simulink model "engineModelF16"  (R2024a)
settings: configuration reference "standardSILConfiguraitonParams" (kept outside this file)
undefined symbols (not defined in the file): engineDataF16, lbf2N, m2ft, parameters, stepSize_s
libraries: simulink x10
settings Model: Creator=jerem  LastModifiedBy=jerem
settings ConfigSetRef: SourceName=standardSILConfiguraitonParams  SourceLocation=Base Workspace

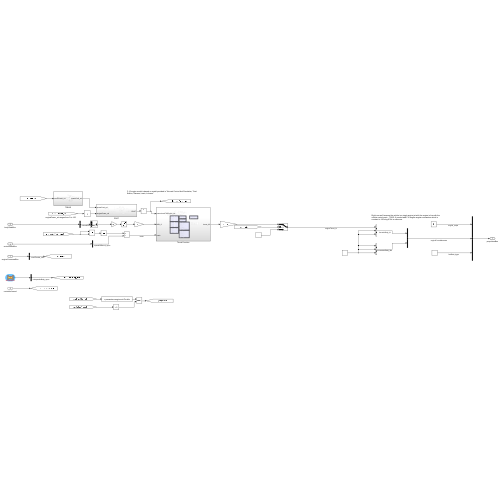
[thumbnail: Simulink's stored preview of the top-level diagram]
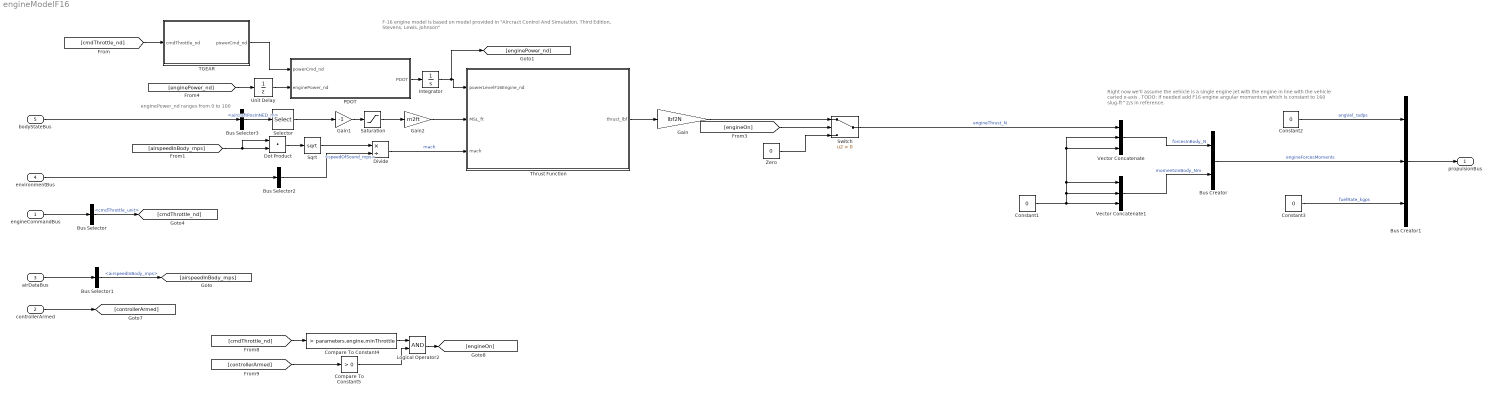
== system engineModelF16 ==
  note: enginePower_nd ranges from 0 to 100
  note: F-16 engine model is based on model provided in "Aircract Control And Simulation, Third Edition, Stevens, Lewis, Johnson"
  note: Right now we'll assume the vehicle is a single engine jet with the engine in line with the vehicle caried x-axis . TODO: If needed add F16 engine angular momentum which is constant to 160 slug-ft^2/s in reference.
  engineCommandBus : Inport  OutDataTypeStr=Bus: EngineCommandBus
  controllerArmed : Inport  Port=2
  airDataBus : Inport  Port=3  OutDataTypeStr=Bus: AirDataBus
  environmentBus : Inport  Port=4  OutDataTypeStr=Bus: EnvironmentBus
  bodyStateBus : Inport  Port=5  OutDataTypeStr=Bus: BodyStateBus
  Bus Creator : BusCreator  Inputs=2
  Bus Creator1 : BusCreator  Inputs=3  OutDataTypeStr=Bus: PropulsionBus
  Bus Selector : BusSelector  OutputSignals=cmdThrottle_unit
  Bus Selector1 : BusSelector  OutputSignals=airspeedInBody_mps
  Bus Selector2 : BusSelector  OutputSignals=AirEnvironment.speedOfSound_mps
  Bus Selector3 : BusSelector  OutputSignals=aircraftPosInNED_m
  Compare To Constant4 : simulink/Logic and Bit Operations/Compare To Constant  relop=>  const=parameters.engine.minThrottle  OutDataTypeStr=boolean
  Compare To Constant5 : simulink/Logic and Bit Operations/Compare To Constant  relop=>  const=0  OutDataTypeStr=boolean
  Constant1 : Constant  Value=0  SampleTime=stepSize_s
  Constant2 : Constant  Value=0  SampleTime=stepSize_s
  Constant3 : Constant  Value=0  SampleTime=stepSize_s
  Divide : Product  Inputs=*/
  Dot Product : DotProduct  OutDataTypeStr=Inherit: Inherit via internal rule
  Gain : Gain  Gain=lbf2N
  Gain1 : Gain  Gain=-1
  Gain2 : Gain  Gain=m2ft
  Integrator : Integrator
  Logical Operator2 : Logic  AllPortsSameDT=off  OutDataTypeStr=boolean
  PDOT : Subsystem
  Saturation : Saturate  UpperLimit=850000  LowerLimit=-1000
  Selector : Selector  InputPortWidth=3  IndexOptions=Index vector (dialog)  Indices=3  OutputSizes=1
  Sqrt : Sqrt
  Switch : Switch  Criteria=u2 > Threshold  SaturateOnIntegerOverflow=off  InputSameDT=off
  TGEAR : Subsystem
  Thrust Function : Subsystem
  Unit Delay : UnitDelay  SampleTime=-1  HasFrameUpgradeWarning=on
  Vector Concatenate : Concatenate  NumInputs=3
  Vector Concatenate1 : Concatenate  NumInputs=3
  Zero : Constant  Value=0  OutDataTypeStr=Inherit: Inherit via back propagation  SampleTime=stepSize_s
  propulsionBus : Outport  OutDataTypeStr=Bus: PropulsionBus
  wires:
  Thrust Function/1(thrust_lbf) -> Gain/1
  Constant1/1 -> Vector Concatenate1/3, Vector Concatenate1/2, Vector Concatenate1/1, Vector Concatenate/3, Vector Concatenate/2
  Vector Concatenate/1 -> Bus Creator/1  "forcesInBody_N"
  Vector Concatenate1/1 -> Bus Creator/2  "momentsInBody_Nm"
  Bus Creator/1 -> Bus Creator1/2  "engineForcesMoments"
  Bus Creator1/1 -> propulsionBus/1
  Constant2/1 -> Bus Creator1/1  "angVel_radps"
  Constant3/1 -> Bus Creator1/3  "fuelRate_kgps"
  Bus Selector/1 -> [cmdThrottle_nd]  "<cmdThrottle_unit>"
  [cmdThrottle_nd] -> Compare To Constant4/1
  engineCommandBus/1 -> Bus Selector/1
  Logical Operator2/1 -> [engineOn]
  controllerArmed/1 -> [controllerArmed]
  airDataBus/1 -> Bus Selector1/1
  Compare To Constant4/1 -> Logical Operator2/1
  Compare To Constant5/1 -> Logical Operator2/2
  [controllerArmed] -> Compare To Constant5/1
  Bus Selector1/1 -> [airspeedInBody_mps]  "<airspeedInBody_mps>"
  Divide/1 -> Thrust Function/3(mach)  "mach"
  environmentBus/1 -> Bus Selector2/1
  Bus Selector2/1 -> Divide/2  "<speedOfSound_mps>"
  bodyStateBus/1 -> Bus Selector3/1
  Bus Selector3/1 -> Selector/1  "<aircraftPosInNED_m>"
  Gain1/1 -> Saturation/1
  Gain2/1 -> Thrust Function/2(MSL_ft)
  Saturation/1 -> Gain2/1
  Selector/1 -> Gain1/1
  [airspeedInBody_mps] -> Dot Product/1, Dot Product/2
  Dot Product/1 -> Sqrt/1
  Sqrt/1 -> Divide/1
  [enginePower_nd] -> Unit Delay/1
  Gain/1 -> Switch/1
  Zero/1 -> Switch/3
  Switch/1 -> Vector Concatenate/1  "engineThrust_N"
  [engineOn] -> Switch/2
  PDOT/1(PDOT) -> Integrator/1
  Integrator/1 -> [enginePower_nd], Thrust Function/1(powerLevelF16Engine_nd)
  Unit Delay/1 -> PDOT/2(enginePower_nd)
  [cmdThrottle_nd] -> TGEAR/1(cmdThrottle_nd)
  TGEAR/1(powerCmd_nd) -> PDOT/1(powerCmd_nd)

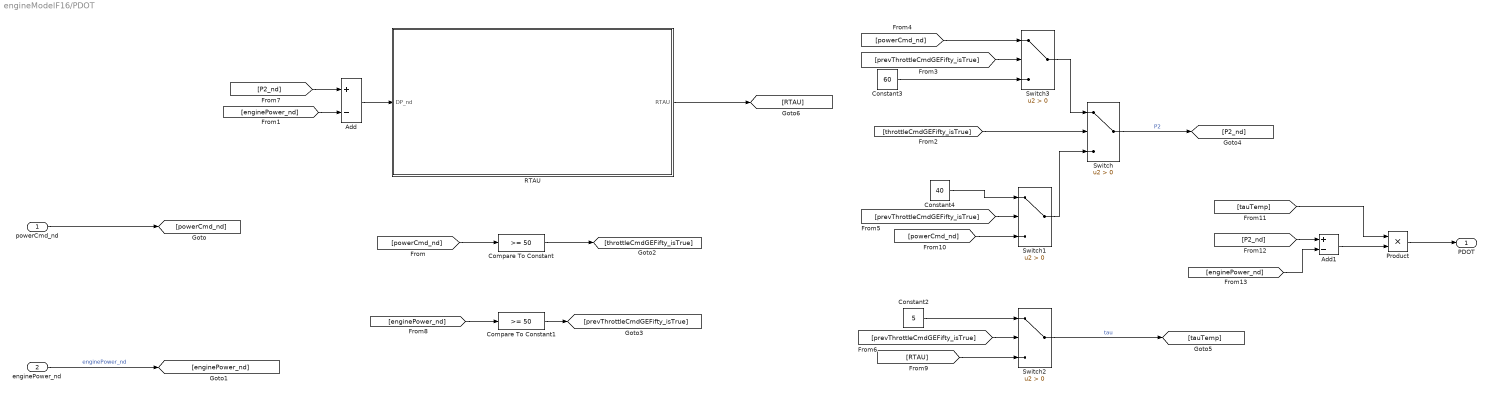
== system engineModelF16/PDOT ==
  powerCmd_nd : Inport
  enginePower_nd : Inport  Port=2
  Add : Sum  Inputs=+-
  Add1 : Sum  Inputs=+-
  Compare To Constant : simulink/Logic and Bit Operations/Compare To Constant  relop=>=  const=50  OutDataTypeStr=boolean
  Compare To Constant1 : simulink/Logic and Bit Operations/Compare To Constant  relop=>=  const=50  OutDataTypeStr=boolean
  Constant2 : Constant  Value=5
  Constant3 : Constant  Value=60
  Constant4 : Constant  Value=40
  Product : Product
  RTAU : Subsystem
  Switch{,1..3} (4 alike) : Switch  Criteria=u2 > Threshold  SaturateOnIntegerOverflow=off  InputSameDT=off
  PDOT : Outport
  wires:
  powerCmd_nd/1 -> [powerCmd_nd]
  enginePower_nd/1 -> [enginePower_nd]  "enginePower_nd"
  [powerCmd_nd] -> Compare To Constant/1
  Compare To Constant/1 -> [throttleCmdGEFifty_isTrue]
  [enginePower_nd] -> Compare To Constant1/1
  Compare To Constant1/1 -> [prevThrottleCmdGEFifty_isTrue]
  [prevThrottleCmdGEFifty_isTrue] -> Switch3/2
  [throttleCmdGEFifty_isTrue] -> Switch/2
  Switch/1 -> [P2_nd]  "P2"
  [prevThrottleCmdGEFifty_isTrue] -> Switch2/2
  Switch2/1 -> [tauTemp]  "tau"
  [P2_nd] -> Add/1
  [enginePower_nd] -> Add/2
  Add/1 -> RTAU/1(DP_nd)
  RTAU/1(RTAU) -> [RTAU]
  Constant2/1 -> Switch2/1
  [RTAU] -> Switch2/3
  [powerCmd_nd] -> Switch3/1
  Switch3/1 -> Switch/1
  Constant3/1 -> Switch3/3
  Switch1/1 -> Switch/3
  [prevThrottleCmdGEFifty_isTrue] -> Switch1/2
  Constant4/1 -> Switch1/1
  [powerCmd_nd] -> Switch1/3
  [P2_nd] -> Add1/1
  [enginePower_nd] -> Add1/2
  Add1/1 -> Product/2
  [tauTemp] -> Product/1
  Product/1 -> PDOT/1

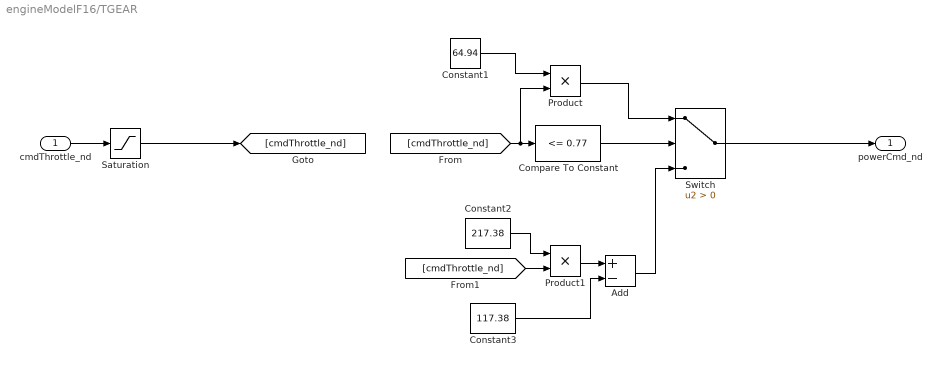
== system engineModelF16/TGEAR ==
  cmdThrottle_nd : Inport
  Add : Sum  Inputs=+-
  Compare To Constant : simulink/Logic and Bit Operations/Compare To Constant  relop=<=  const=0.77  OutDataTypeStr=boolean
  Constant1 : Constant  Value=64.94
  Constant2 : Constant  Value=217.38
  Constant3 : Constant  Value=117.38
  Product : Product
  Product1 : Product
  Saturation : Saturate  UpperLimit=1  LowerLimit=0
  Switch : Switch  Criteria=u2 > Threshold  SaturateOnIntegerOverflow=off  InputSameDT=off
  powerCmd_nd : Outport
  wires:
  cmdThrottle_nd/1 -> Saturation/1
  [cmdThrottle_nd] -> Compare To Constant/1, Product/2
  Compare To Constant/1 -> Switch/2
  Product/1 -> Switch/1
  Constant1/1 -> Product/1
  [cmdThrottle_nd] -> Product1/2
  Constant2/1 -> Product1/1
  Product1/1 -> Add/1
  Constant3/1 -> Add/2
  Add/1 -> Switch/3
  Switch/1 -> powerCmd_nd/1
  Saturation/1 -> [cmdThrottle_nd]

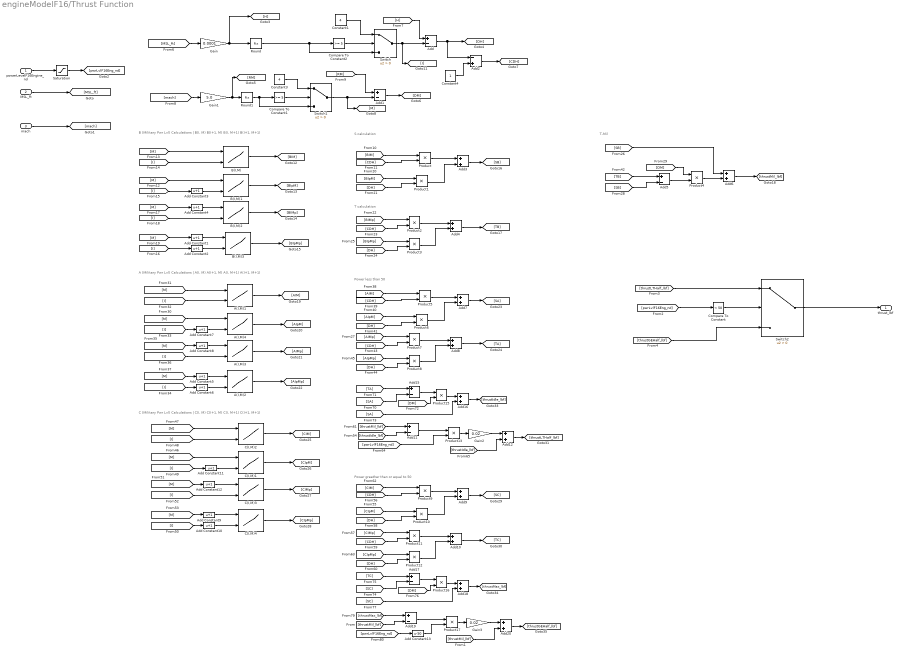
== system engineModelF16/Thrust Function ==
  note: S calculation
  note: B (Military Pwr Lvl) Calculations | B(I, M) B(I+1, M) B(I, M+1) B(I+1, M+1)
  note: T calculation
  note: T-Mil
  note: Power less than 50
  note: A (Military Pwr Lvl) Calculations | A(I, M) A(I+1, M) A(I, M+1) A(I+1, M+1)
  note: C (Military Pwr Lvl) Calculations | C(I, M) C(I+1, M) C(I, M+1) C(I+1, M+1)
  note: Power greather than or equal to 50
  powerLevelF16Engine_nd : Inport  OutDataTypeStr=double
  MSL_ft : Inport  Port=2
  mach : Inport  Port=3
  A(I,M){1..4} (4 alike) : Lookup_n-D  BreakpointsForDimension1=engineDataF16.machBkpts  BreakpointsForDimension2=engineDataF16.altitudeBkpts_ft  Table=engineDataF16.thrustIdle_lbf  ExtrapMethod=Clip  DiagnosticForOutOfRangeInput=Warning  InternalRulePriority=Speed  RndMeth=Simplest
      settings: InputPortMap=u0,u1
  Add{,1,5,11,15,17,19} (7 alike) : Sum  Inputs=+-
  Add Constant{1..12} (12 alike) : Bias  Bias=1  SaturateOnIntegerOverflow=off
  Add Constant13 : Bias  Bias=-50  SaturateOnIntegerOverflow=off
  Add{3..4,6..10,12,16,18,20} (11 alike) : Sum
  Add2 : Sum  Inputs=-+
  B(I,M){,1..3} (4 alike) : Lookup_n-D  BreakpointsForDimension1=engineDataF16.machBkpts  BreakpointsForDimension2=engineDataF16.altitudeBkpts_ft  Table=engineDataF16.thrustMilitary_lbf  ExtrapMethod=Clip  DiagnosticForOutOfRangeInput=Warning  InternalRulePriority=Speed  RndMeth=Simplest
      settings: InputPortMap=u0,u1
  C(I,M){1..4} (4 alike) : Lookup_n-D  BreakpointsForDimension1=engineDataF16.machBkpts  BreakpointsForDimension2=engineDataF16.altitudeBkpts_ft  Table=engineDataF16.thrustMax_lbf  ExtrapMethod=Clip  DiagnosticForOutOfRangeInput=Warning  InternalRulePriority=Speed  RndMeth=Simplest
      settings: InputPortMap=u0,u1
  Compare To Constant : simulink/Logic and Bit Operations/Compare To Constant  relop=<  const=50  OutDataTypeStr=boolean
  Compare To Constant1 : simulink/Logic and Bit Operations/Compare To Constant  relop=>=  const=5  OutDataTypeStr=boolean
  Compare To Constant2 : simulink/Logic and Bit Operations/Compare To Constant  relop=>=  const=5  OutDataTypeStr=boolean
  Constant1 : Constant  Value=4
  Constant3 : Constant  Value=4
  Constant4 : Constant
  Gain : Gain  Gain=0.0001
  Gain1 : Gain  Gain=5.0
  Gain2 : Gain  Gain=0.02
  Gain3 : Gain  Gain=0.02
  Product{,1..13,15..17} (17 alike) : Product
  Round : Rounding  Operator=fix
  Round1 : Rounding  Operator=fix
  Saturation : Saturate  UpperLimit=100  LowerLimit=0
  Switch : Switch  Criteria=u2 > Threshold  SaturateOnIntegerOverflow=off  InputSameDT=off
  Switch1 : Switch  Criteria=u2 > Threshold  SaturateOnIntegerOverflow=off  InputSameDT=off
  Switch2 : Switch  Criteria=u2 > Threshold  SaturateOnIntegerOverflow=off  InputSameDT=off
  thrust_lbf : Outport
  wires:
  powerLevelF16Engine_nd/1 -> Saturation/1
  MSL_ft/1 -> [MSL_ft]
  mach/1 -> [mach]
  [MSL_ft] -> Gain/1
  Gain/1 -> [H], Round/1
  Round/1 -> Compare To Constant2/1, Switch/3
  Compare To Constant2/1 -> Switch/2
  Constant1/1 -> Switch/1
  [H] -> Add/1
  Switch/1 -> [I], Add/2
  Add/1 -> Add2/1, [DH]
  [mach] -> Gain1/1
  Round1/1 -> Compare To Constant1/1, Switch1/3
  Compare To Constant1/1 -> Switch1/2
  Constant3/1 -> Switch1/1
  Gain1/1 -> [RM], Round1/1
  Switch1/1 -> [M], Add1/2
  [RM] -> Add1/1
  Add1/1 -> [DM]
  Constant4/1 -> Add2/2
  Add2/1 -> [CDH]
  [BIM] -> Product/1
  [CDH] -> Product/2
  Product/1 -> Add3/1
  [I] -> Add Constant3/1
  [M] -> Add Constant4/1
  [I] -> Add Constant2/1
  [M] -> Add Constant1/1
  B(I,M)/1 -> [BIM]
  B(I,M)1/1 -> [BIpM]
  B(I,M)2/1 -> [BIMp]
  B(I,M)3/1 -> [BIpMp]
  [BIpM] -> Product1/1
  [DH] -> Product1/2
  Product1/1 -> Add3/2
  Add3/1 -> [SB]
  [BIMp] -> Product2/1
  [CDH] -> Product2/2
  Product2/1 -> Add4/1
  [DH] -> Product3/2
  [BIpMp] -> Product3/1
  Product3/1 -> Add4/2
  Add4/1 -> [TB]
  [TB] -> Add5/1
  [SB] -> Add5/2
  Add5/1 -> Product4/2
  [DM] -> Product4/1
  Product4/1 -> Add6/2
  [SB] -> Add6/1
  Add6/1 -> [thrustMil_lbf]
  [M] -> Add Constant8/1
  [I] -> Add Constant6/1
  A(I,M)3/1 -> [AIMp]
  [I] -> Add Constant7/1
  A(I,M)2/1 -> [AIpMp]
  [M] -> Add Constant5/1
  A(I,M)1/1 -> [AIM]
  A(I,M)4/1 -> [AIpM]
  [CDH] -> Product5/2
  Product5/1 -> Add7/1
  [AIM] -> Product5/1
  [DH] -> Product6/2
  Product6/1 -> Add7/2
  [AIpM] -> Product6/1
  Add7/1 -> [SA]
  [DH] -> Product8/2
  [AIpMp] -> Product8/1
  Product7/1 -> Add8/1
  [AIMp] -> Product7/1
  Product8/1 -> Add8/2
  [CDH] -> Product7/2
  Add8/1 -> [TA]
  C(I,M)4/1 -> [CIpMp]
  C(I,M)1/1 -> [CIpM]
  [M] -> Add Constant9/1
  C(I,M)2/1 -> [CIM]
  C(I,M)3/1 -> [CIMp]
  [M] -> Add Constant12/1
  [I] -> Add Constant11/1
  [I] -> Add Constant10/1
  Product10/1 -> Add9/2
  Add9/1 -> [SC]
  [CIpM] -> Product10/1
  Product11/1 -> Add10/1
  Add10/1 -> [TC]
  Product12/1 -> Add10/2
  [DH] -> Product12/2
  [DH] -> Product10/2
  [CIM] -> Product9/1
  [CIMp] -> Product11/1
  Product9/1 -> Add9/1
  [CIpMp] -> Product12/1
  [CDH] -> Product9/2
  [CDH] -> Product11/2
  [TA] -> Add15/1
  [SA] -> Add15/2
  Add15/1 -> Product15/1
  [DM] -> Product15/2
  Product15/1 -> Add16/1
  [SA] -> Add16/2
  Add16/1 -> [thrustIdle_lbf]
  [thrustMil_lbf] -> Add11/1
  [thrustIdle_lbf] -> Add11/2
  Add11/1 -> Product13/1
  [pwrLvlF16Eng_nd] -> Product13/2
  Product13/1 -> Gain2/1
  Gain2/1 -> Add12/1
  [thrustIdle_lbf] -> Add12/2
  Add12/1 -> [thrustLTHalf_lbf]
  Add17/1 -> Product16/1
  [DM] -> Product16/2
  Add18/1 -> [thrustMax_lbf]
  [TC] -> Add17/1
  [SC] -> Add18/2
  [SC] -> Add17/2
  Product16/1 -> Add18/1
  [thrustMil_lbf] -> Add19/2
  Add20/1 -> [thrustGEHalf_lbf]
  [thrustMil_lbf] -> Add20/2
  Gain3/1 -> Add20/1
  [pwrLvlF16Eng_nd] -> Add Constant13/1
  Add19/1 -> Product17/1
  Product17/1 -> Gain3/1
  [thrustMax_lbf] -> Add19/1
  Add Constant13/1 -> Product17/2
  [pwrLvlF16Eng_nd] -> Compare To Constant/1
  Saturation/1 -> [pwrLvlF16Eng_nd]
  Compare To Constant/1 -> Switch2/2
  [thrustGEHalf_lbf] -> Switch2/3
  [thrustLTHalf_lbf] -> Switch2/1
  Switch2/1 -> thrust_lbf/1
  [M] -> B(I,M)/1
  [I] -> B(I,M)/2
  Add Constant3/1 -> B(I,M)1/2
  [M] -> B(I,M)1/1
  Add Constant4/1 -> B(I,M)2/1
  [I] -> B(I,M)2/2
  Add Constant2/1 -> B(I,M)3/2
  Add Constant1/1 -> B(I,M)3/1
  [M] -> A(I,M)1/1
  [I] -> A(I,M)1/2
  Add Constant7/1 -> A(I,M)4/2
  [M] -> A(I,M)4/1
  Add Constant8/1 -> A(I,M)3/1
  [I] -> A(I,M)3/2
  [M] -> C(I,M)2/1
  [I] -> C(I,M)2/2
  Add Constant11/1 -> C(I,M)1/2
  [M] -> C(I,M)1/1
  Add Constant12/1 -> C(I,M)3/1
  [I] -> C(I,M)3/2
  Add Constant10/1 -> C(I,M)4/2
  Add Constant9/1 -> C(I,M)4/1
  Add Constant5/1 -> A(I,M)2/1
  Add Constant6/1 -> A(I,M)2/2

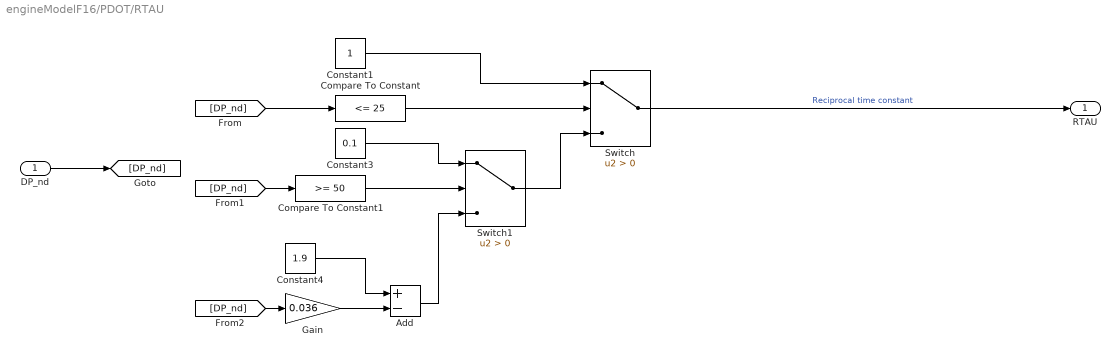
== system engineModelF16/PDOT/RTAU ==
  DP_nd : Inport
  Add : Sum  Inputs=+-
  Compare To Constant : simulink/Logic and Bit Operations/Compare To Constant  relop=<=  const=25  OutDataTypeStr=boolean
  Compare To Constant1 : simulink/Logic and Bit Operations/Compare To Constant  relop=>=  const=50  OutDataTypeStr=boolean
  Constant1 : Constant
  Constant3 : Constant  Value=0.1
  Constant4 : Constant  Value=1.9
  Gain : Gain  Gain=0.036
  Switch : Switch  Criteria=u2 > Threshold  SaturateOnIntegerOverflow=off  InputSameDT=off
  Switch1 : Switch  Criteria=u2 > Threshold  SaturateOnIntegerOverflow=off  InputSameDT=off
  RTAU : Outport
  wires:
  DP_nd/1 -> [DP_nd]
  [DP_nd] -> Compare To Constant/1
  Switch/1 -> RTAU/1  "Reciprocal time constant"
  Constant1/1 -> Switch/1
  [DP_nd] -> Compare To Constant1/1
  Compare To Constant1/1 -> Switch1/2
  Constant3/1 -> Switch1/1
  Switch1/1 -> Switch/3
  [DP_nd] -> Gain/1
  Gain/1 -> Add/2
  Constant4/1 -> Add/1
  Add/1 -> Switch1/3
  Compare To Constant/1 -> Switch/2
